simulink model "Trapezoid_profil"  (R2021a)
settings: Solver=VariableStepAuto  StartTime=0.0  StopTime=10  RelTol=1e-3
settings Model: Creator=serkan  LastModifiedBy=serkan

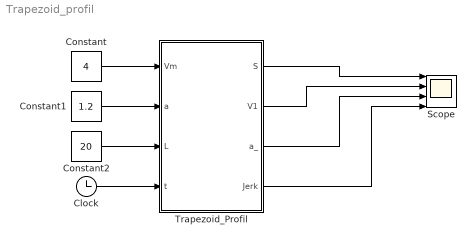
== system Trapezoid_profil ==
  Clock : Clock
  Constant : Constant  Value=4
  Constant1 : Constant  Value=1.2
  Constant2 : Constant  Value=20
  Scope : Scope  NumInputPorts=4
  Trapezoid_Profil : Subsystem
  wires:
  Constant/1 -> Trapezoid_Profil/1(Vm)
  Constant1/1 -> Trapezoid_Profil/2(a)
  Constant2/1 -> Trapezoid_Profil/3(L)
  Clock/1 -> Trapezoid_Profil/4(t)
  Trapezoid_Profil/1(S) -> Scope/1
  Trapezoid_Profil/2(V1) -> Scope/2
  Trapezoid_Profil/3(a_) -> Scope/3
  Trapezoid_Profil/4(Jerk) -> Scope/4

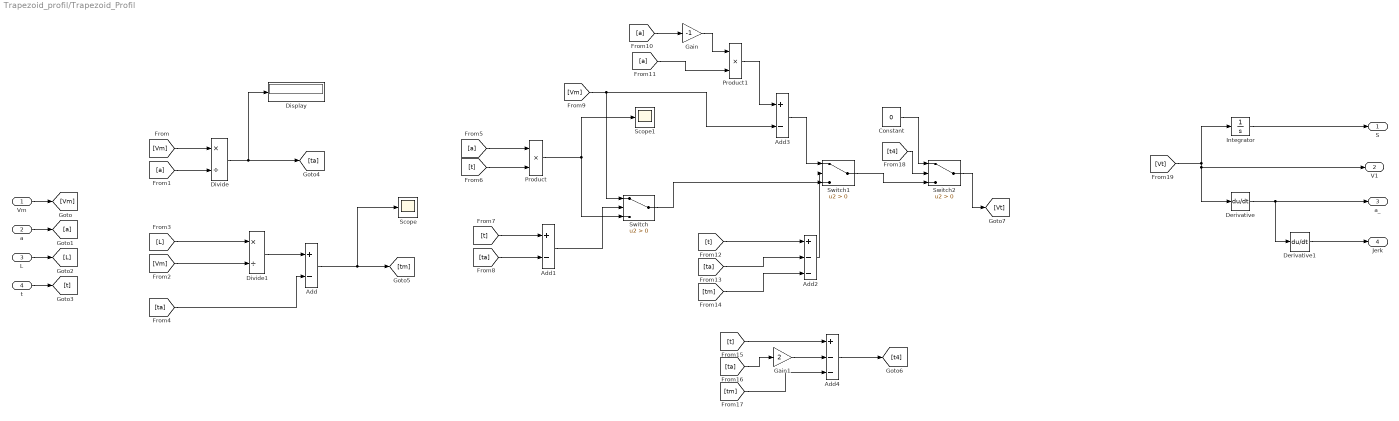
== system Trapezoid_profil/Trapezoid_Profil ==
  Vm : Inport
  a : Inport  Port=2
  L : Inport  Port=3
  t : Inport  Port=4
  Add : Sum  Inputs=+-
  Add1 : Sum  Inputs=+-
  Add2 : Sum  Inputs=+--
  Add3 : Sum  Inputs=+-
  Add4 : Sum  Inputs=+--
  Constant : Constant  Value=0
  Derivative : Derivative
  Derivative1 : Derivative
  Display : Display
  Divide : Product  Inputs=*/
  Divide1 : Product  Inputs=*/
  Gain : Gain  Gain=-1
  Gain1 : Gain  Gain=2
  Integrator : Integrator
  Product : Product
  Product1 : Product
  Scope : Scope
  Scope1 : Scope
  Switch : Switch  Criteria=u2 > Threshold
  Switch1 : Switch  Criteria=u2 > Threshold
  Switch2 : Switch  Criteria=u2 > Threshold
  S : Outport
  V1 : Outport  Port=2
  a_ : Outport  Port=3
  Jerk : Outport  Port=4
  wires:
  [Vm] -> Divide/1
  Product/1 -> Switch/3, Scope1/1
  [a] -> Divide/2
  Vm/1 -> [Vm]
  Divide1/1 -> Add/1
  [ta] -> Add/2
  Add/1 -> Scope/1, [tm]
  [Vm] -> Divide1/2
  Divide/1 -> [ta], Display/1
  [a] -> Product/1
  [t] -> Product/2
  t/1 -> [t]
  L/1 -> [L]
  a/1 -> [a]
  [L] -> Divide1/1
  [t] -> Add1/1
  [ta] -> Add1/2
  Add1/1 -> Switch/2
  Switch/1 -> Switch1/3
  [Vm] -> Add3/2, Switch/1
  [a] -> Gain/1
  Gain/1 -> Product1/1
  [a] -> Product1/2
  Product1/1 -> Add3/1
  Add3/1 -> Switch1/1
  [t] -> Add2/1
  [ta] -> Add2/2
  [tm] -> Add2/3
  Add2/1 -> Switch1/2
  [t] -> Add4/1
  [tm] -> Add4/3
  Add4/1 -> [t4]
  [ta] -> Gain1/1
  Gain1/1 -> Add4/2
  Constant/1 -> Switch2/1
  [t4] -> Switch2/2
  Switch1/1 -> Switch2/3
  Switch2/1 -> [Vt]
  [Vt] -> Derivative/1, V1/1, Integrator/1
  Integrator/1 -> S/1
  Derivative/1 -> Derivative1/1, a_/1
  Derivative1/1 -> Jerk/1
